simulink model "Model_2"  (R2019b)
settings: Solver=VariableStepAuto  StartTime=0.0  StopTime=10.0  RelTol=1e-3
values from neighbouring files (symbols this model uses):
  A = [0, 1, 0, 0 ... (first row only)    [Pendulum_2.m]
  B = [0; (I+m*l^2)/q; 0; (m*l)/q]    [Pendulum_2.m]
  C = [1 0 0 0]    [Pendulum_2.m]
  k_d = acker(Ad,Bd,Pole_Shift_d)    [Pendulum_2.m]
  X0 = [0; 3*pi/180; 0; 0]    [Pendulum_2.m]
settings Model: Creator=jose_  LastModifiedBy=jose_

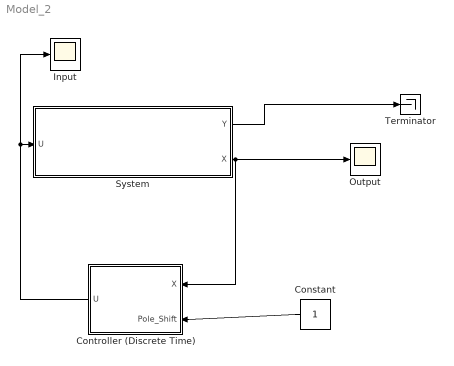
== system Model_2 ==
  Constant : Constant
  Controller (Discrete Time) : Subsystem
  "Input " : Scope
  "Output " : Scope
  System : Subsystem
  Terminator : Terminator
  wires:
  System/1(Y) -> Terminator/1
  Constant/1 -> Controller (Discrete Time)/2(Pole_Shift)
  System/2(X) -> Controller (Discrete Time)/1(X), "Output "/1
  Controller (Discrete Time)/1(U) -> "Input "/1, System/1(U)

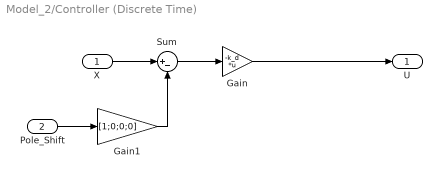
== system Model_2/Controller (Discrete Time) ==
  X : Inport
  Pole_Shift : Inport  Port=2
  Gain : Gain  Gain=-k_d  Multiplication=Matrix(K*u)
  Gain1 : Gain  Gain=[1;0;0;0]
  Sum : Sum  Inputs=|+-
  U : Outport
  wires:
  Gain/1 -> U/1
  X/1 -> Sum/1
  Sum/1 -> Gain/1
  Pole_Shift/1 -> Gain1/1
  Gain1/1 -> Sum/2

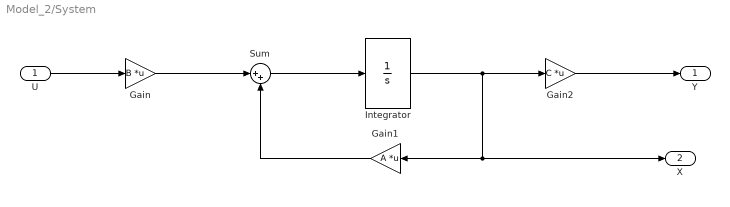
== system Model_2/System ==
  U : Inport
  Gain : Gain  Gain=B  Multiplication=Matrix(K*u)
  Gain1 : Gain  Gain=A  Multiplication=Matrix(K*u)
  Gain2 : Gain  Gain=C  Multiplication=Matrix(K*u)
  Integrator : Integrator  InitialCondition=X0
  Sum : Sum  Inputs=|++
  Y : Outport
  X : Outport  Port=2
  wires:
  Sum/1 -> Integrator/1
  Gain/1 -> Sum/1
  Gain1/1 -> Sum/2
  Integrator/1 -> Gain2/1, X/1, Gain1/1
  U/1 -> Gain/1
  Gain2/1 -> Y/1
